simulink model "simulacion_cascada"  (R2019a)
settings: Solver=VariableStepAuto  StartTime=0.0  StopTime=650  RelTol=1e-3
libraries: cstblocks x17
settings Model: Creator=Juan P Velandia  LastModifiedBy=Juan P Velandia

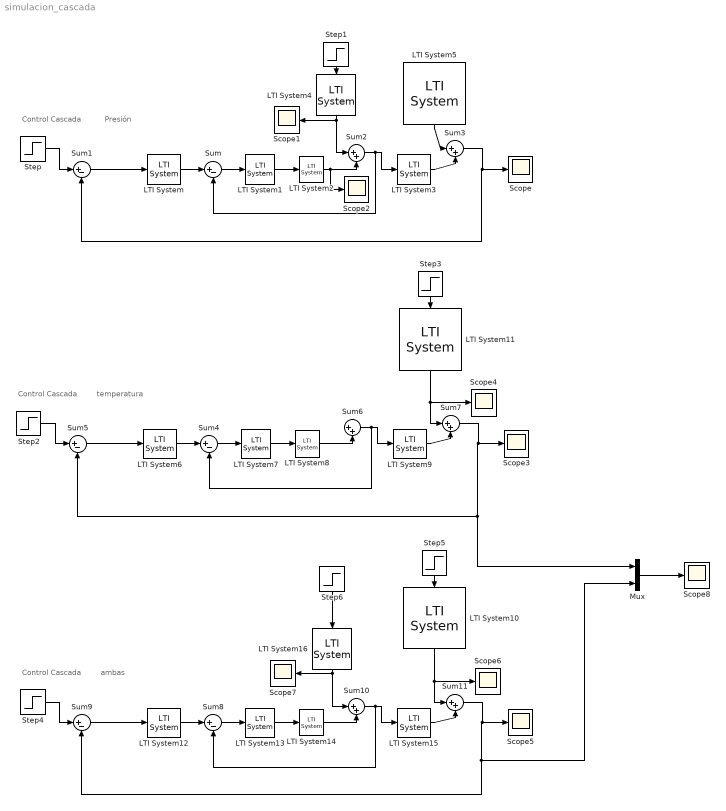
== system simulacion_cascada ==
  note: temperatura
  note: Presión
  note: Control Cascada
  note: Control Cascada
  note: Control Cascada
  note: ambas
  LTI System : cstblocks/LTI System  sys=C2  IC=[]
  LTI System1 : cstblocks/LTI System  sys=C1  IC=[]
  LTI System10 : cstblocks/LTI System  sys=P_temperatura  IC=[]
  LTI System11 : cstblocks/LTI System  sys=P_temperatura  IC=[]
  LTI System12 : cstblocks/LTI System  sys=C2  IC=[]
  LTI System13 : cstblocks/LTI System  sys=C1  IC=[]
  LTI System14 : cstblocks/LTI System  sys=G1  IC=[]
  LTI System15 : cstblocks/LTI System  sys=G2  IC=[]
  LTI System16 : cstblocks/LTI System  sys=P_presion  IC=[]
  LTI System2 : cstblocks/LTI System  sys=G1  IC=[]
  LTI System3 : cstblocks/LTI System  sys=G2  IC=[]
  LTI System4 : cstblocks/LTI System  sys=P_presion  IC=[]
  LTI System5 : cstblocks/LTI System  sys=P_temperatura  IC=[]
  LTI System6 : cstblocks/LTI System  sys=C2  IC=[]
  LTI System7 : cstblocks/LTI System  sys=C1  IC=[]
  LTI System8 : cstblocks/LTI System  sys=G1  IC=[]
  LTI System9 : cstblocks/LTI System  sys=G2  IC=[]
  Mux : Mux  Inputs=2
  Scope{,1..8} (9 alike) : Scope
  Step : Step  After=80  SampleTime=0
  Step1 : Step  Time=400  After=150  SampleTime=0
  Step2 : Step  After=80  SampleTime=0
  Step3 : Step  Time=400  After=30  SampleTime=0
  Step4 : Step  After=80  SampleTime=0
  Step5 : Step  Time=400  After=30  SampleTime=0
  Step6 : Step  Time=400  After=150  SampleTime=0
  Sum{,1,4..5,8..9} (6 alike) : Sum  Inputs=|+-
  Sum{2..3,6..7,10..11} (6 alike) : Sum  Inputs=|++
  wires:
  LTI System/1 -> Sum/1
  Sum/1 -> LTI System1/1
  LTI System1/1 -> LTI System2/1
  Sum1/1 -> LTI System/1
  Step/1 -> Sum1/1
  Sum2/1 -> Sum/2, LTI System3/1
  LTI System2/1 -> Sum2/2, Scope2/1
  LTI System3/1 -> Sum3/2
  Sum3/1 -> Sum1/2, Scope/1
  LTI System4/1 -> Sum2/1, Scope1/1
  LTI System5/1 -> Sum3/1
  Step1/1 -> LTI System4/1
  Sum7/1 -> Mux/1, Sum5/2, Scope3/1
  Step2/1 -> Sum5/1
  LTI System11/1 -> Scope4/1, Sum7/1
  LTI System9/1 -> Sum7/2
  LTI System7/1 -> LTI System8/1
  LTI System6/1 -> Sum4/1
  LTI System8/1 -> Sum6/2
  Sum5/1 -> LTI System6/1
  Sum6/1 -> Sum4/2, LTI System9/1
  Sum4/1 -> LTI System7/1
  Step3/1 -> LTI System11/1
  LTI System15/1 -> Sum11/2
  LTI System10/1 -> Scope6/1, Sum11/1
  Step4/1 -> Sum9/1
  Sum11/1 -> Mux/2, Sum9/2, Scope5/1
  Sum10/1 -> Sum8/2, LTI System15/1
  Sum8/1 -> LTI System13/1
  Sum9/1 -> LTI System12/1
  LTI System13/1 -> LTI System14/1
  LTI System14/1 -> Sum10/2
  LTI System12/1 -> Sum8/1
  Step5/1 -> LTI System10/1
  LTI System16/1 -> Sum10/1, Scope7/1
  Step6/1 -> LTI System16/1
  Mux/1 -> Scope8/1
